simulink model "EKF_model_ToComplete"  (R2022b)
settings: Solver=VariableStepAuto  StartTime=0.0  StopTime=40000  RelTol=1e-3  EnableMultiTasking=on
InitFcn:
  | T = 0.1;
  | R0=0.24;
  | R1=0.1;
  | C1=920;
  | Cn=2.6
undefined symbols (not defined in the file): sigbuilder_block
settings Model: Creator=yahia  LastModifiedBy=M._Yahia
settings SolverCC: AlgebraicLoopSolver=TrustRegion
settings DataIOCC: ReturnWorkspaceOutputs=off
settings OptimizationCC: LifeSpan=inf
settings DebuggingCC: UnconnectedInputMsg=warning  UnconnectedOutputMsg=warning  UnconnectedLineMsg=warning  SFUnexpectedBacktrackingDiag=warning  SFNoUnconditionalDefaultTransitionDiag=warning  SFMachineParentedDataDiag=warning  ArithmeticOperatorsInVariantConditions=warning
settings ModelReferenceCC: EnableRefExpFcnMdlSchedulingChecks=on
settings SFSimCC: SimUseLocalCustomCode=off  CustomCodeUndefinedFunction=UseInterfaceOnly
settings RTWCC: RTWUseLocalCustomCode=off  DLArmComputeVersion=19.05
settings CodeAppCC: StateflowObjectComments=on
settings GRTTargetCC: TargetLangStandard=C89/C90 (ANSI)
settings ConfigComp: CovMetricSettings=dw  CovSaveCumulativeToWorkspaceVar=on  CovSaveSingleToWorkspaceVar=on  CovExternalEMLEnable=off

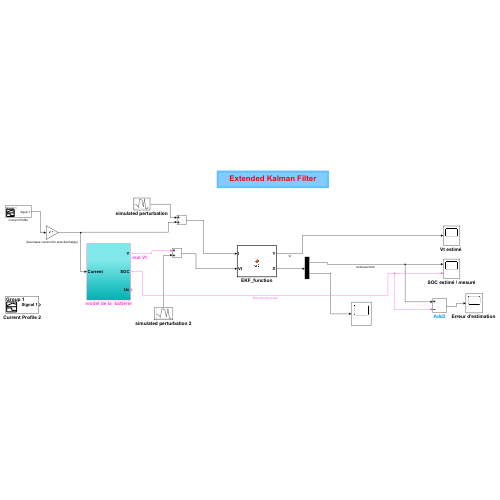
[thumbnail: Simulink's stored preview of the top-level diagram]
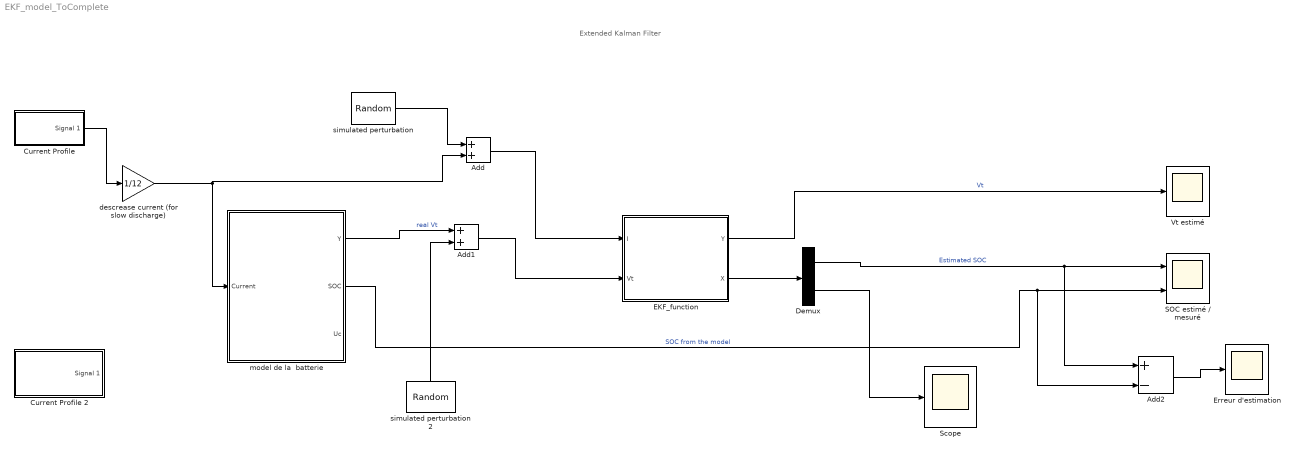
== system EKF_model_ToComplete ==
  note: Extended Kalman Filter
  Add : Sum
  Add1 : Sum
  Add2 : Sum  Inputs=+-
  Current Profile : Subsystem  Tag=STV Subsys  LoadFcn=sigbuilder_block('load');  StartFcn=sigbuilder_block('start');  StopFcn=sigbuilder_block('stop');  ClipboardFcn=sigbuilder_block('clipboard');  mask(Sigbuilder block){tuvar=[0:10]}
      mask help: Simulink:masks:SigbuilderBlock_MD
      mask init:
      | if ~strcmp(get_param(bdroot(gcbh),'SimulationStatus'),'stopped') tuvar = sigbuilder_block('maskInit'); end
      settings: CopyFcn=sigbuilder_block('copy');  DeleteFcn=sigbuilder_block('delete');  ModelCloseFcn=sigbuilder_block('modelClose');  PreSaveFcn=sigbuilder_block('preSave');  PauseFcn=sigbuilder_block('pause');  ContinueFcn=sigbuilder_block('continue');  NameChangeFcn=sigbuilder_block('namechange');  OpenFcn=sigbuilder_block('open',[5.4 5.4 1141.2 580.8 ]);  CloseFcn=sigbuilder_block('close');
      mask Display: plot(0, 0, 100, 100,[2, 2, 32, 32, 2], [68, 8, 8, 68, 68],[32, 2], [38, 38], [32, 19, 2],[53, 60, 44], [32, 17, 17, 2],[16, 16, 31, 31]);txt = getActiveGroup(gcbh);text(2, 100, txt,'verticalAlignment', 'top');
  Current Profile 2 : Subsystem  Tag=STV Subsys  LoadFcn=sigbuilder_block('load');  StartFcn=sigbuilder_block('start');  StopFcn=sigbuilder_block('stop');  ClipboardFcn=sigbuilder_block('clipboard');  mask(Sigbuilder block){tuvar=[0:10]}
      mask help: Simulink:masks:SigbuilderBlock_MD
      mask init:
      | if ~strcmp(get_param(bdroot(gcbh),'SimulationStatus'),'stopped') tuvar = sigbuilder_block('maskInit'); end
      settings: CopyFcn=sigbuilder_block('copy');  DeleteFcn=sigbuilder_block('delete');  ModelCloseFcn=sigbuilder_block('modelClose');  PreSaveFcn=sigbuilder_block('preSave');  PauseFcn=sigbuilder_block('pause');  ContinueFcn=sigbuilder_block('continue');  NameChangeFcn=sigbuilder_block('namechange');  OpenFcn=sigbuilder_block('open',[117.75 190.5 614.25 322.5 ]);  CloseFcn=sigbuilder_block('close');
      mask Display: plot(0, 0, 100, 100,[2, 2, 32, 32, 2], [68, 8, 8, 68, 68],[32, 2], [38, 38], [32, 19, 2],[53, 60, 44], [32, 17, 17, 2],[16, 16, 31, 31]);txt = getActiveGroup(gcbh);text(2, 100, txt,'verticalAlignment', 'top');
  Demux : Demux  Outputs=2
  EKF_function : MATLAB Function  TreatAsAtomicUnit=on
  "Erreur d'estimation " : Scope
  SOC estimé / mesuré : Scope  NumInputPorts=2
  Scope : Scope
  "Vt estimé " : Scope
  descrease current (for slow discharge) : Gain  Gain=1/12
  model de la  batterie : Subsystem
  simulated perturbation : RandomNumber  Variance=0.01  SampleTime=0.1
  simulated perturbation 2 : RandomNumber  Variance=00.01  SampleTime=0.1
  wires:
  simulated perturbation/1 -> Add/1
  model de la  batterie/1(Y) -> Add1/1  "real Vt"
  simulated perturbation 2/1 -> Add1/2
  Add/1 -> EKF_function/1(I)
  Add1/1 -> EKF_function/2(Vt)
  Demux/1 -> Add2/1, SOC estimé / mesuré/1  "Estimated SOC"
  model de la  batterie/2(SOC) -> Add2/2, SOC estimé / mesuré/2  "SOC from the model"
  EKF_function/2(X) -> Demux/1
  EKF_function/1(Y) -> "Vt estimé "/1  "Vt"
  Add2/1 -> "Erreur d'estimation "/1
  descrease current (for slow discharge)/1 -> model de la  batterie/1(Current), Add/2
  Demux/2 -> Scope/1
  Current Profile/1(Signal 1) -> descrease current (for slow discharge)/1

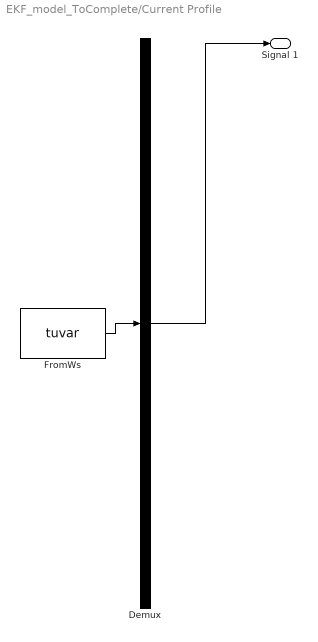
== system EKF_model_ToComplete/Current Profile ==
  Demux : Demux  Tag=STV Demux  Outputs=1
      settings: DisplayOption=none
  FromWs : FromWorkspace  Tag=STV FromWs  VariableName=tuvar
      SigBuilderData=|
      | common.afterFinalStr = 'Extrapolate'
      | common.sampleTime = 0
      | dataSet.timeRange = [0 40000]
      | dataSet.name = 'Group 1'
      | sbobj.Groups.Name = 'Group 1'
      | sbobj.Groups.Signals.Name = 'Signal 1'
      | sbobj.Groups.Signals.XData = [0 1000 1000 2000 2000 3000 3000 4000 4000 5000 5000 6000 6000 7000 7000 8000 8000 9000 9000 10000 10000 11000 11000 12000 12000 13000 13000 14000 14000 15000 15000 16000 16000 17000 17000 18000 18000 19000 19000 20000 20000 21000 21000 22000 22000 23000 23000 24000 24000 25000 25000 26000 26000 27000 27000 28000 28000 29000 29000 30000 30000 31000 31000 32000 32000 33000 33000 34000 34000 35000 35000 36000 36000 37000 37000 38000 38000 39000 39000 40000]
      | sbobj.Groups.Signals.YData = [0 0 -10 -10 0 0 -10 -10 0 0 -10 -10 0 0 -10 -10 0 0 -10 -10 0 0 -10 -10 0 0 -10 -10 0 0 -10 -10 0 0 -10 -10 0 0 -10 -10 0 0 10 10 0 0 10 10 0 0 10 10 0 0 10 10 0 0 10 10 0 0 10 10 0 0 10 10 0 0 10 10 0 0 10 10 0 0 10 10]
      | sbobj.Groups.TimeRange = [0 40000]
  Signal 1 : Outport  Tag=STV Outport
  wires:
  Demux/1 -> Signal 1/1
  FromWs/1 -> Demux/1

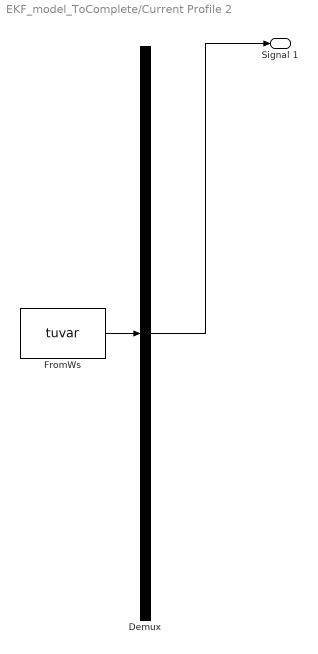
== system EKF_model_ToComplete/Current Profile 2 ==
  Demux : Demux  Tag=STV Demux  Outputs=1
      settings: DisplayOption=none
  FromWs : FromWorkspace  Tag=STV FromWs  VariableName=tuvar
      SigBuilderData=|
      | common.afterFinalStr = 'Extrapolate'
      | common.sampleTime = 0
      | dataSet.timeRange = [0 24500]
      | dataSet.name = 'Group 1'
      | sbobj.Groups.Name = 'Group 1'
      | sbobj.Groups.Signals.Name = 'Signal 1'
      | sbobj.Groups.Signals.XData = [0 24500]
      | sbobj.Groups.Signals.YData = [-0.38 -0.38]
      | sbobj.Groups.TimeRange = [0 24500]
  Signal 1 : Outport  Tag=STV Outport
  wires:
  Demux/1 -> Signal 1/1
  FromWs/1 -> Demux/1

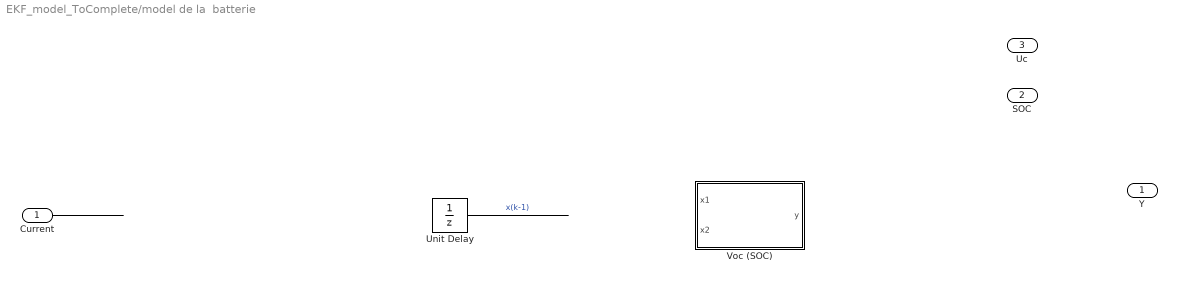
== system EKF_model_ToComplete/model de la  batterie ==
  Current : Inport
  Unit Delay : UnitDelay  InitialCondition=[1;0]  SampleTime=0.1  HasFrameUpgradeWarning=on
  Voc (SOC) : MATLAB Function  TreatAsAtomicUnit=on
  Y : Outport
  SOC : Outport  Port=2
  Uc : Outport  Port=3
  wires:
  ? -> Unit Delay/1  "x(k)"
  Current/1 -> ?
  Unit Delay/1 -> ?  "x(k-1)"
  ? -> Y/1  "C * x(k-1) + B*U"
  ? -> SOC/1
  ? -> Uc/1

== matlab function EKF_model_ToComplete/model de la  batterie/Voc (SOC) ==
  data: x1 input; y output; x2 input
function y = J(x1,x2)
%#codegen

y = ....;

== matlab function EKF_model_ToComplete/EKF_function ==
  data: I input; Y output; X output; Vt input
function [Y,X] = fcn2(I,Vt)

%============ info to consider !!! ========================
%==========================================================

% P > 0: State Covariance Matrix, is a square matrix of 2x2 (number of states)
% Q > 0: Process Noise Covariance Matrix, uncertainty or noise introduced by
% the system's dynamics : 2 x 2 square matrix
% R > 0: Measurement Noise Covariance Matrix : uncertainty or noise in the
% measurements. one output (Vt) so R is just a positivenumber in our case

R0 = 0.24;
R1 = 0.1;
C1 = 920;
Cn = 2.6 ;
T = 0.1;

persistent P Xhat A B C D Q R 
% initialisation 
if isempty(P);

sum = 0;

% ======== intialize state and covariance matrices

Xhat = .... ;
   P = .... ;
   Q = .... ;
   R = ..... ;
end

% ===================  calculate A, B, D matices 
A = ... ;
B = .... ;
D = ... ;

% ==== calculate the new Xhat matrix and then calculate C matrix obtained
% using jacobian derivation (first-order partial derivatives of Vt function)
 
Xhat = A*Xhat + B*I;
Z = Xhat(1); % here for simplicity we take Z as the actual SOC value (first element of the state matrix) 

C = [ 'obtained function', 1];

P = ;

K = ;
% calculate error err = Vt - "estimated Vt" 
 
% complete the other code parts 

% at the end, the output is the actual Y output using the new Xhat
